simulink model "chokedOrifice"  (Simulink 10.0)
settings: Solver=VariableStepAuto  StartTime=0.0  StopTime=10.0  RelTol=1e-3
undefined symbols (not defined in the file or in its folder): sigbuilder_block
libraries: nesl_utility x6, fl_lib x5, sh_lib x1
(part 2 of 2)

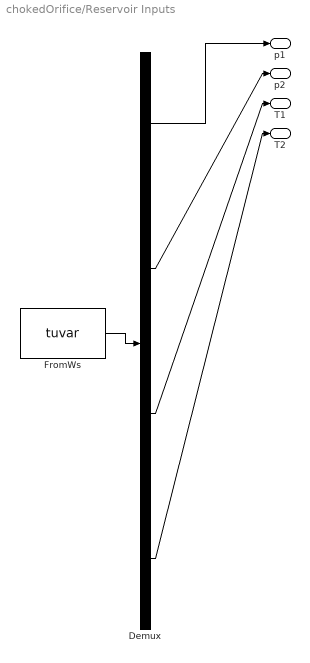
== system chokedOrifice/Reservoir Inputs ==
  Demux : Demux  Tag=STV Demux
  FromWs : FromWorkspace  Tag=STV FromWs  VariableName=tuvar  SampleTime=0  SigBuilderData=DataTag0  VnvData=DataTag1
      SigBuilderData=|
      | common.afterFinalStr = 'Extrapolate'
      | common.sampleTime = 0
      | dataSet.timeRange = [0 10]
      | dataSet.name = 'Group 1'
      | sbobj.Groups.Name = 'Group 1'
      | sbobj.Groups.Signals(1).Name = 'p1'
      | sbobj.Groups.Signals(1).XData = [0 6 9 10]
      | sbobj.Groups.Signals(1).YData = [0.5 0.5 0.8 0.8]
      | sbobj.Groups.Signals(2).Name = 'p2'
      | sbobj.Groups.Signals(2).XData = [0 1 5 10]
      | sbobj.Groups.Signals(2).YData = [0.5 0.5 0.2 0.2]
      | sbobj.Groups.Signals(3).Name = 'T1'
      | sbobj.Groups.Signals(3).XData = [0 10]
      | sbobj.Groups.Signals(3).YData = [300 300]
      | sbobj.Groups.Signals(4).Name = 'T2'
      | sbobj.Groups.Signals(4).XData = [0 10]
      | sbobj.Groups.Signals(4).YData = [300 300]
  p1 : Outport  Tag=STV Outport  VectorParamsAs1DForOutWhenUnconnected=off
  p2 : Outport  Tag=STV Outport  Port=2  VectorParamsAs1DForOutWhenUnconnected=off
  T1 : Outport  Tag=STV Outport  Port=3  VectorParamsAs1DForOutWhenUnconnected=off
  T2 : Outport  Tag=STV Outport  Port=4  VectorParamsAs1DForOutWhenUnconnected=off
  wires:
  Demux/1 -> p1/1
  FromWs/1 -> Demux/1
  Demux/2 -> p2/1
  Demux/3 -> T1/1
  Demux/4 -> T2/1

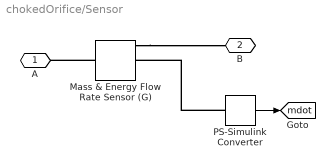
== system chokedOrifice/Sensor ==
  Mass & Energy Flow Rate Sensor (G) : fl_lib/Gas/Sensors/Mass & Energy Flow Rate Sensor (G)
      settings: SourceProductName=Simscape  SourceProductBaseCode=SS  InternalSimscapePortConfiguration="{\"Bottom\":[],\"Left\":[{\"id\":\"A\",\"label\":\"A\",\"type\":\"foundation.gas.gas\"}],\"Right\":[{\"id\":\"B\",\"label\":\"B\",\"type\":\"foundation.gas.gas\"},{\"id\":\"M\",\"label\":\"M\",\"type\":\"output\"},{\"id\":\"PHI\",\"label\":\"Phi\",\"type\":\"output\"}],\"Top\":[]}"
  PS-Simulink Converter : nesl_utility/PS-Simulink Converter  PhysicalDomain=network_engine_domain  SubClassName=ps_output  LeftPortType=input  RightPortType=output  PseudoPeriodic=off  Frequencies=[]  Unit=kg/s  AffineConversion=off
  A : PMIOPort  Side=Left
  B : PMIOPort  Port=2  Side=Right
  tag scope: mdot=global
  wires:
  PS-Simulink Converter/1 -> [mdot]
  connections:
  PS-Simulink Converter/LConn1 -- Mass & Energy Flow Rate Sensor (G)/RConn2
  Mass & Energy Flow Rate Sensor (G)/LConn1 -- A/RConn1
  Mass & Energy Flow Rate Sensor (G)/RConn1 -- B/RConn1
